simulink model "lab_5_sim2"  (R2018a)
settings: Solver=ode45  StartTime=0.0  StopTime=20  RelTol=1e-3  AbsTol=1e-6  EnableMultiTasking=on
undefined symbols (not defined in the file): a, b, c, d, du, t0, t1, u0, x0, x10
settings Model: Creator=LAB320-1552  LastModifiedBy=johnb
settings SolverCC: AutoScaleAbsTol=off
settings DataIOCC: LimitDataPoints=on  SaveFormat=Array
settings OptimizationCC: LifeSpan=inf
settings DebuggingCC: UnderspecifiedInitializationDetection=Classic  MergeDetectMultiDrivingBlocksExec=none  StateNameClashWarn=warning  SFUnexpectedBacktrackingDiag=warning  SFNoUnconditionalDefaultTransitionDiag=warning  SFExecutionAtInitializationDiag=none
settings HardwareCC: ProdBitPerPointer=32  ProdBitPerSizeT=32  ProdBitPerPtrDiffT=32  ProdLargestAtomicFloat=None  ProdIntDivRoundTo=Undefined  ProdEndianess=Unspecified  ProdWordSize=32  ProdHWDeviceType=32-bit Generic
settings ModelReferenceCC: PropagateSignalLabelsOutOfModel=off
settings CodeAppCC: StateflowObjectComments=on
settings GRTTargetCC: TargetLangStandard=C89/C90 (ANSI)  GeneratePreprocessorConditionals=Disable all
settings ConfigComp: CovMetricSettings=dw  CovHtmlReporting=on  CovSaveCumulativeToWorkspaceVar=on  CovSaveSingleToWorkspaceVar=on  CovExternalEMLEnable=off

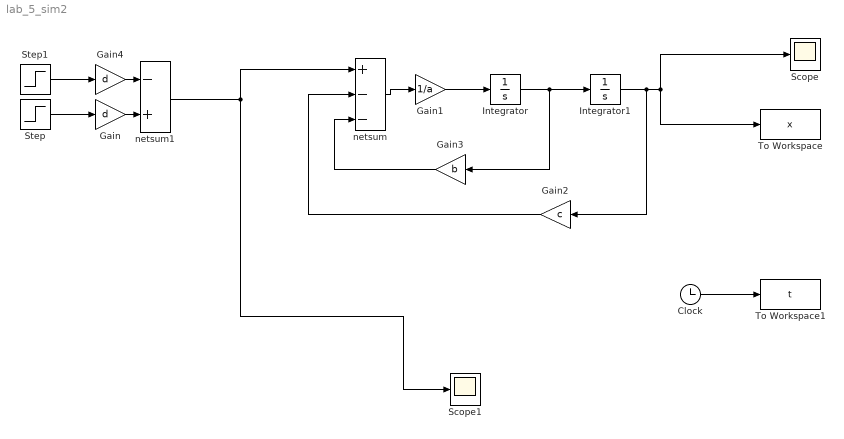
== system lab_5_sim2 ==
  Clock : Clock
  Gain : Gain  Gain=d
  Gain1 : Gain  Gain=1/a
  Gain2 : Gain  Gain=c
  Gain3 : Gain  Gain=b
  Gain4 : Gain  Gain=d
  Integrator : Integrator  InitialCondition=x10
  Integrator1 : Integrator  InitialCondition=x0
  Scope : Scope
  Scope1 : Scope
  Step : Step  Time=t0  Before=u0  After=u0+du  SampleTime=1
  Step1 : Step  After=u0+du  SampleTime=t1
  To Workspace : ToWorkspace  VariableName=x  SampleTime=-1
  To Workspace1 : ToWorkspace  VariableName=t  SampleTime=-1
  netsum : Sum  Inputs=+--  SaturateOnIntegerOverflow=on  InputSameDT=on  OutDataTypeStr=Inherit: Same as first input
  netsum1 : Sum  Inputs=-+  SaturateOnIntegerOverflow=on  InputSameDT=on  OutDataTypeStr=Inherit: Same as first input
  wires:
  Step/1 -> Gain/1
  netsum/1 -> Gain1/1
  Integrator/1 -> Gain3/1, Integrator1/1
  Integrator1/1 -> Gain2/1, Scope/1, To Workspace/1
  Gain2/1 -> netsum/2
  Clock/1 -> To Workspace1/1
  Gain1/1 -> Integrator/1
  Step1/1 -> Gain4/1
  Gain/1 -> netsum1/2
  Gain4/1 -> netsum1/1
  netsum1/1 -> Scope1/1, netsum/1
  Gain3/1 -> netsum/3
